simulink model "SecRwRtStLtwdRtwdIsPosChk"  (R2018b)
settings: Solver=FixedStepDiscrete  StartTime=0.0  StopTime=10.0  FixedStep=0.01  RelTol=1e-3
undefined symbols (not defined in the file or in its folder): KeSMSuSecRwStLwdRwdPosDelta_Val, KeSMSuSecRwStLwdRwdPosTolr_Val
libraries: StIsPosChkLib x9, simulink x5
settings Model: Creator=sn2xws  LastModifiedBy=sn2xws
settings DataIOCC: SaveFormat=StructureWithTime
settings OptimizationCC: DefaultParameterBehavior=Inlined  EnhancedBackFolding=on  PassReuseOutputArgsAs=Individual arguments  ZeroExternalMemoryAtStartup=off  ZeroInternalMemoryAtStartup=off  OptimizeBlockOrder=speed  DifferentSizesBufferReuse=on  OptimizationCustomize=off
settings DebuggingCC: ParameterTunabilityLossMsg=error
settings ModelReferenceCC: ModelReferenceNumInstancesAllowed=Single
settings SFSimCC: MATLABDynamicMemAlloc=off
settings RTWCC: SystemTargetFile=autosar.tlc  GenCodeOnly=on  TemplateMakefile=ert_default_tmf  Description=AUTOSAR  GenerateReport=on  IncludeHyperlinkInReport=on  LaunchReport=on  GenerateTraceInfo=on  GenerateTraceReport=on  GenerateTraceReportSl=on  GenerateTraceReportSf=on  GenerateTraceReportEml=on
settings CodeAppCC: ForceParamTrailComments=on  IgnoreCustomStorageClasses=off  OperatorAnnotations=on  SimulinkDataObjDesc=on  SFDataObjDesc=on  InsertBlockDesc=on
settings STFCustomTargetCC: TargetLangStandard=C99 (ISO)  MultiwordLength=256  ParMdlRefBuildCompliant=on  CompOptLevelCompliant=on  IncludeMdlTerminateFcn=off  CombineOutputUpdateFcns=on  SuppressErrorStatus=on  ERTCustomFileBanners=on  SupportNonFinite=off  SupportComplex=off  SupportContinuousTime=off  SupportNonInlinedSFcns=off  RemoveResetFunc=on  MATLABClassNameForMDSCustomization=Simulink.SoftwareTarget.ERTCustomization  AutosarCompliant=on  UseToolchainInfoCompliant=on  LookupTableObjectStructAxisOrder=2,1,3,4,...  LUTObjectStructOrderEvenSpacing=Size,Table,Breakpoints  SystemTargetFile=autosar.tlc
settings ERTTargetCC: TargetLangStandard=C99 (ISO)  ConcurrentExecutionCompliant=off  IncludeMdlTerminateFcn=off  SuppressErrorStatus=on  SupportNonFinite=off  SupportComplex=off  ModelStepFunctionPrototypeControlCompliant=off  CPPClassGenCompliant=off  AutosarCompliant=on  LookupTableObjectStructAxisOrder=2,1,3,4,...  LUTObjectStructOrderEvenSpacing=Size,Table,Breakpoints  InlinedParameterPlacement=NonHierarchical  ERTCustomFileTemplate=example_file_process.tlc  ERTFilePackagingFormat=Compact

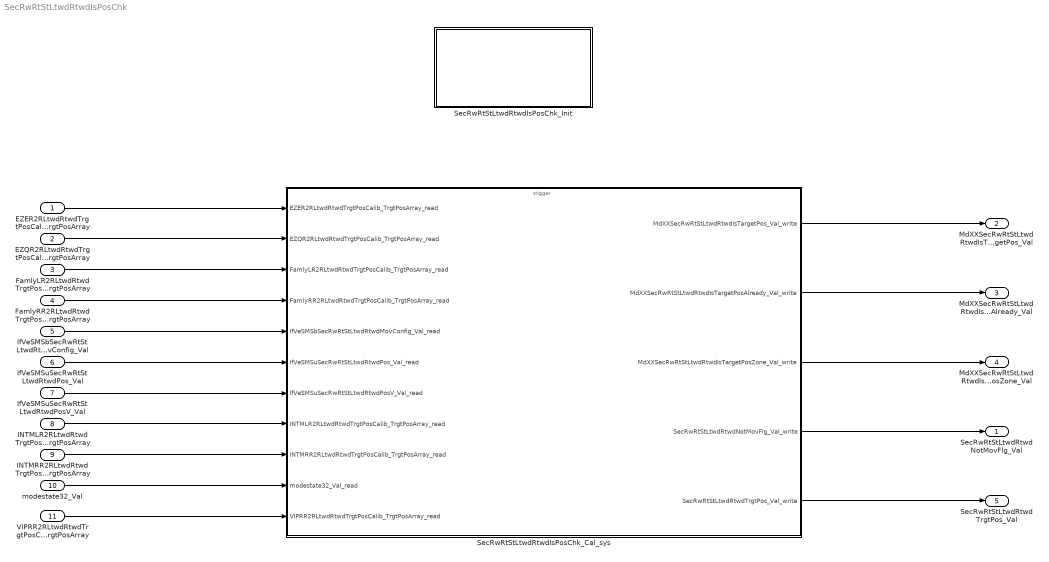
== system SecRwRtStLtwdRtwdIsPosChk ==
  EZER2RLtwdRtwdTrgtPosCalib_TrgtPosArray : Inport  Description=|  OutDataTypeStr=uint16  PortDimensions=3
      | 0:Pos
      | 1:Max
      | 2:Min
  EZQR2RLtwdRtwdTrgtPosCalib_TrgtPosArray : Inport  Description=|  Port=2  OutDataTypeStr=uint16  PortDimensions=3
      | 0:Pos
      | 1:Max
      | 2:Min
  FamlyLR2RLtwdRtwdTrgtPosCalib_TrgtPosArray : Inport  Description=|  Port=3  OutDataTypeStr=uint16  PortDimensions=3
      | 0:Pos
      | 1:Max
      | 2:Min
  FamlyRR2RLtwdRtwdTrgtPosCalib_TrgtPosArray : Inport  Description=|  Port=4  OutDataTypeStr=uint16  PortDimensions=3
      | 0:Pos
      | 1:Max
      | 2:Min
  IfVeSMSbSecRwRtStLtwdRtwdMovConfig_Val : Inport  Port=5  OutDataTypeStr=boolean  PortDimensions=1
  IfVeSMSuSecRwRtStLtwdRtwdPos_Val : Inport  Port=6  OutDataTypeStr=uint16  PortDimensions=1
  IfVeSMSuSecRwRtStLtwdRtwdPosV_Val : Inport  Port=7  OutDataTypeStr=boolean  PortDimensions=1
  INTMLR2RLtwdRtwdTrgtPosCalib_TrgtPosArray : Inport  Description=|  Port=8  OutDataTypeStr=uint16  PortDimensions=3
      | 0:Pos
      | 1:Max
      | 2:Min
  INTMRR2RLtwdRtwdTrgtPosCalib_TrgtPosArray : Inport  Description=|  Port=9  OutDataTypeStr=uint16  PortDimensions=3
      | 0:Pos
      | 1:Max
      | 2:Min
  modestate32_Val : Inport  Port=10  OutDataTypeStr=uint32  PortDimensions=1
  VIPRR2RLtwdRtwdTrgtPosCalib_TrgtPosArray : Inport  Description=|  Port=11  OutDataTypeStr=uint16  PortDimensions=3
      | 0:Pos
      | 1:Max
      | 2:Min
  SecRwRtStLtwdRtwdIsPosChk_Cal_sys : Subsystem
  SecRwRtStLtwdRtwdIsPosChk_Init : Subsystem
  SecRwRtStLtwdRtwdNotMovFlg_Val : Outport  OutDataTypeStr=boolean  PortDimensions=1
  MdXXSecRwRtStLtwdRtwdIsTargetPos_Val : Outport  Port=2  OutDataTypeStr=uint32  PortDimensions=1
  MdXXSecRwRtStLtwdRtwdIsTargetPosAlready_Val : Outport  Port=3  OutDataTypeStr=uint32  PortDimensions=1
  MdXXSecRwRtStLtwdRtwdIsTargetPosZone_Val : Outport  Port=4  OutDataTypeStr=uint32  PortDimensions=1
  SecRwRtStLtwdRtwdTrgtPos_Val : Outport  Port=5  OutDataTypeStr=uint16  PortDimensions=1
  wires:
  EZER2RLtwdRtwdTrgtPosCalib_TrgtPosArray/1 -> SecRwRtStLtwdRtwdIsPosChk_Cal_sys/1(EZER2RLtwdRtwdTrgtPosCalib_TrgtPosArray_read)
  EZQR2RLtwdRtwdTrgtPosCalib_TrgtPosArray/1 -> SecRwRtStLtwdRtwdIsPosChk_Cal_sys/2(EZQR2RLtwdRtwdTrgtPosCalib_TrgtPosArray_read)
  FamlyLR2RLtwdRtwdTrgtPosCalib_TrgtPosArray/1 -> SecRwRtStLtwdRtwdIsPosChk_Cal_sys/3(FamlyLR2RLtwdRtwdTrgtPosCalib_TrgtPosArray_read)
  FamlyRR2RLtwdRtwdTrgtPosCalib_TrgtPosArray/1 -> SecRwRtStLtwdRtwdIsPosChk_Cal_sys/4(FamlyRR2RLtwdRtwdTrgtPosCalib_TrgtPosArray_read)
  IfVeSMSbSecRwRtStLtwdRtwdMovConfig_Val/1 -> SecRwRtStLtwdRtwdIsPosChk_Cal_sys/5(IfVeSMSbSecRwRtStLtwdRtwdMovConfig_Val_read)
  IfVeSMSuSecRwRtStLtwdRtwdPos_Val/1 -> SecRwRtStLtwdRtwdIsPosChk_Cal_sys/6(IfVeSMSuSecRwRtStLtwdRtwdPos_Val_read)
  IfVeSMSuSecRwRtStLtwdRtwdPosV_Val/1 -> SecRwRtStLtwdRtwdIsPosChk_Cal_sys/7(IfVeSMSuSecRwRtStLtwdRtwdPosV_Val_read)
  INTMLR2RLtwdRtwdTrgtPosCalib_TrgtPosArray/1 -> SecRwRtStLtwdRtwdIsPosChk_Cal_sys/8(INTMLR2RLtwdRtwdTrgtPosCalib_TrgtPosArray_read)
  INTMRR2RLtwdRtwdTrgtPosCalib_TrgtPosArray/1 -> SecRwRtStLtwdRtwdIsPosChk_Cal_sys/9(INTMRR2RLtwdRtwdTrgtPosCalib_TrgtPosArray_read)
  modestate32_Val/1 -> SecRwRtStLtwdRtwdIsPosChk_Cal_sys/10(modestate32_Val_read)
  VIPRR2RLtwdRtwdTrgtPosCalib_TrgtPosArray/1 -> SecRwRtStLtwdRtwdIsPosChk_Cal_sys/11(VIPRR2RLtwdRtwdTrgtPosCalib_TrgtPosArray_read)
  SecRwRtStLtwdRtwdIsPosChk_Cal_sys/1(MdXXSecRwRtStLtwdRtwdIsTargetPos_Val_write) -> MdXXSecRwRtStLtwdRtwdIsTargetPos_Val/1
  SecRwRtStLtwdRtwdIsPosChk_Cal_sys/2(MdXXSecRwRtStLtwdRtwdIsTargetPosAlready_Val_write) -> MdXXSecRwRtStLtwdRtwdIsTargetPosAlready_Val/1
  SecRwRtStLtwdRtwdIsPosChk_Cal_sys/3(MdXXSecRwRtStLtwdRtwdIsTargetPosZone_Val_write) -> MdXXSecRwRtStLtwdRtwdIsTargetPosZone_Val/1
  SecRwRtStLtwdRtwdIsPosChk_Cal_sys/4(SecRwRtStLtwdRtwdNotMovFlg_Val_write) -> SecRwRtStLtwdRtwdNotMovFlg_Val/1
  SecRwRtStLtwdRtwdIsPosChk_Cal_sys/5(SecRwRtStLtwdRtwdTrgtPos_Val_write) -> SecRwRtStLtwdRtwdTrgtPos_Val/1

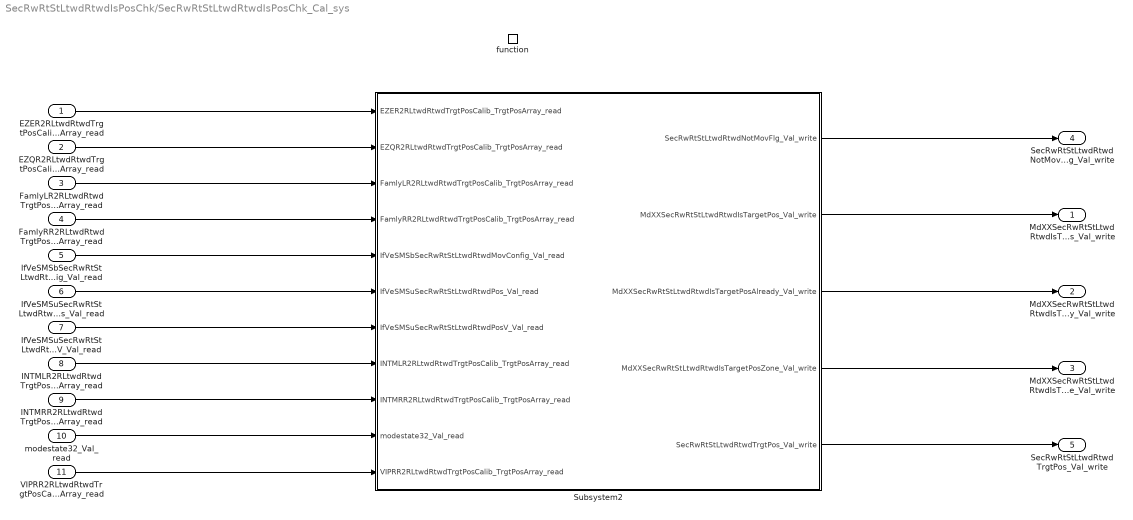
== system SecRwRtStLtwdRtwdIsPosChk/SecRwRtStLtwdRtwdIsPosChk_Cal_sys ==
  EZER2RLtwdRtwdTrgtPosCalib_TrgtPosArray_read : Inport
  EZQR2RLtwdRtwdTrgtPosCalib_TrgtPosArray_read : Inport  Port=2
  FamlyLR2RLtwdRtwdTrgtPosCalib_TrgtPosArray_read : Inport  Port=3
  FamlyRR2RLtwdRtwdTrgtPosCalib_TrgtPosArray_read : Inport  Port=4
  IfVeSMSbSecRwRtStLtwdRtwdMovConfig_Val_read : Inport  Port=5
  IfVeSMSuSecRwRtStLtwdRtwdPos_Val_read : Inport  Port=6
  IfVeSMSuSecRwRtStLtwdRtwdPosV_Val_read : Inport  Port=7
  INTMLR2RLtwdRtwdTrgtPosCalib_TrgtPosArray_read : Inport  Port=8
  INTMRR2RLtwdRtwdTrgtPosCalib_TrgtPosArray_read : Inport  Port=9
  modestate32_Val_read : Inport  Port=10
  VIPRR2RLtwdRtwdTrgtPosCalib_TrgtPosArray_read : Inport  Port=11
  function : TriggerPort  TriggerType=function-call  IsSimulinkFunction=on  FunctionName=SecRwRtStLtwdRtwdIsPosChk_Cal  VariantControl=(inherit)
  Subsystem2 : Subsystem
  MdXXSecRwRtStLtwdRtwdIsTargetPos_Val_write : Outport
      settings: EnsureOutportIsVirtual=on
  MdXXSecRwRtStLtwdRtwdIsTargetPosAlready_Val_write : Outport  Port=2
      settings: EnsureOutportIsVirtual=on
  MdXXSecRwRtStLtwdRtwdIsTargetPosZone_Val_write : Outport  Port=3
      settings: EnsureOutportIsVirtual=on
  SecRwRtStLtwdRtwdNotMovFlg_Val_write : Outport  Port=4
      settings: EnsureOutportIsVirtual=on
  SecRwRtStLtwdRtwdTrgtPos_Val_write : Outport  Port=5
      settings: EnsureOutportIsVirtual=on
  wires:
  EZER2RLtwdRtwdTrgtPosCalib_TrgtPosArray_read/1 -> Subsystem2/1(EZER2RLtwdRtwdTrgtPosCalib_TrgtPosArray_read)
  EZQR2RLtwdRtwdTrgtPosCalib_TrgtPosArray_read/1 -> Subsystem2/2(EZQR2RLtwdRtwdTrgtPosCalib_TrgtPosArray_read)
  FamlyLR2RLtwdRtwdTrgtPosCalib_TrgtPosArray_read/1 -> Subsystem2/3(FamlyLR2RLtwdRtwdTrgtPosCalib_TrgtPosArray_read)
  FamlyRR2RLtwdRtwdTrgtPosCalib_TrgtPosArray_read/1 -> Subsystem2/4(FamlyRR2RLtwdRtwdTrgtPosCalib_TrgtPosArray_read)
  IfVeSMSbSecRwRtStLtwdRtwdMovConfig_Val_read/1 -> Subsystem2/5(IfVeSMSbSecRwRtStLtwdRtwdMovConfig_Val_read)
  IfVeSMSuSecRwRtStLtwdRtwdPos_Val_read/1 -> Subsystem2/6(IfVeSMSuSecRwRtStLtwdRtwdPos_Val_read)
  IfVeSMSuSecRwRtStLtwdRtwdPosV_Val_read/1 -> Subsystem2/7(IfVeSMSuSecRwRtStLtwdRtwdPosV_Val_read)
  INTMLR2RLtwdRtwdTrgtPosCalib_TrgtPosArray_read/1 -> Subsystem2/8(INTMLR2RLtwdRtwdTrgtPosCalib_TrgtPosArray_read)
  INTMRR2RLtwdRtwdTrgtPosCalib_TrgtPosArray_read/1 -> Subsystem2/9(INTMRR2RLtwdRtwdTrgtPosCalib_TrgtPosArray_read)
  modestate32_Val_read/1 -> Subsystem2/10(modestate32_Val_read)
  VIPRR2RLtwdRtwdTrgtPosCalib_TrgtPosArray_read/1 -> Subsystem2/11(VIPRR2RLtwdRtwdTrgtPosCalib_TrgtPosArray_read)
  Subsystem2/1(SecRwRtStLtwdRtwdNotMovFlg_Val_write) -> SecRwRtStLtwdRtwdNotMovFlg_Val_write/1
  Subsystem2/2(MdXXSecRwRtStLtwdRtwdIsTargetPos_Val_write) -> MdXXSecRwRtStLtwdRtwdIsTargetPos_Val_write/1
  Subsystem2/3(MdXXSecRwRtStLtwdRtwdIsTargetPosAlready_Val_write) -> MdXXSecRwRtStLtwdRtwdIsTargetPosAlready_Val_write/1
  Subsystem2/4(MdXXSecRwRtStLtwdRtwdIsTargetPosZone_Val_write) -> MdXXSecRwRtStLtwdRtwdIsTargetPosZone_Val_write/1
  Subsystem2/5(SecRwRtStLtwdRtwdTrgtPos_Val_write) -> SecRwRtStLtwdRtwdTrgtPos_Val_write/1

== system SecRwRtStLtwdRtwdIsPosChk/SecRwRtStLtwdRtwdIsPosChk_Init ==
  Event Listener : EventListener  EventName=reset

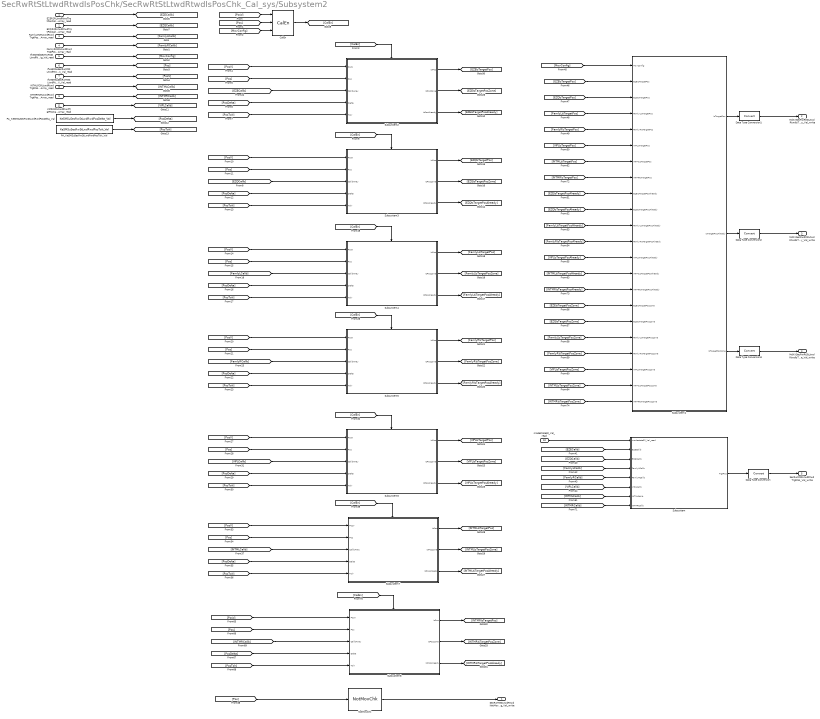
== system SecRwRtStLtwdRtwdIsPosChk/SecRwRtStLtwdRtwdIsPosChk_Cal_sys/Subsystem2 ==
  EZER2RLtwdRtwdTrgtPosCalib_TrgtPosArray_read : Inport
  EZQR2RLtwdRtwdTrgtPosCalib_TrgtPosArray_read : Inport  Port=2
  FamlyLR2RLtwdRtwdTrgtPosCalib_TrgtPosArray_read : Inport  Port=3
  FamlyRR2RLtwdRtwdTrgtPosCalib_TrgtPosArray_read : Inport  Port=4
  IfVeSMSbSecRwRtStLtwdRtwdMovConfig_Val_read : Inport  Port=5
  IfVeSMSuSecRwRtStLtwdRtwdPos_Val_read : Inport  Port=6
  IfVeSMSuSecRwRtStLtwdRtwdPosV_Val_read : Inport  Port=7
  INTMLR2RLtwdRtwdTrgtPosCalib_TrgtPosArray_read : Inport  Port=8
  INTMRR2RLtwdRtwdTrgtPosCalib_TrgtPosArray_read : Inport  Port=9
  modestate32_Val_read : Inport  Port=10
  VIPRR2RLtwdRtwdTrgtPosCalib_TrgtPosArray_read : Inport  Port=11
  CalEn : StIsPosChkLib/CalEn  SystemSampleTime=-1
  Data Type Conversion{,1..3} (4 alike) : DataTypeConversion
  NotMovChk : StIsPosChkLib/NotMovChk  SystemSampleTime=-1
  PA_KeSMSuSecRwStLwdRwdPosDelta_Val : Constant  Value=KeSMSuSecRwStLwdRwdPosDelta_Val
  PA_KeSMSuSecRwStLwdRwdPosTolr_Val : Constant  Value=KeSMSuSecRwStLwdRwdPosTolr_Val
  Subsystem : Subsystem
  Subsystem1 : Subsystem
  Subsystem2 : Subsystem
  Subsystem3 : Subsystem
  Subsystem4 : Subsystem
  Subsystem5 : Subsystem
  Subsystem6 : Subsystem
  Subsystem7 : Subsystem
  Subsystem8 : Subsystem
  SecRwRtStLtwdRtwdNotMovFlg_Val_write : Outport
      settings: EnsureOutportIsVirtual=on
  MdXXSecRwRtStLtwdRtwdIsTargetPos_Val_write : Outport  Port=2
      settings: EnsureOutportIsVirtual=on
  MdXXSecRwRtStLtwdRtwdIsTargetPosAlready_Val_write : Outport  Port=3
      settings: EnsureOutportIsVirtual=on
  MdXXSecRwRtStLtwdRtwdIsTargetPosZone_Val_write : Outport  Port=4
      settings: EnsureOutportIsVirtual=on
  SecRwRtStLtwdRtwdTrgtPos_Val_write : Outport  Port=5
      settings: EnsureOutportIsVirtual=on
  wires:
  [PosTolr] -> Subsystem7/5(Tolr)
  Subsystem6/1(IsPos) -> [VIPLIsTargetPos]
  [INTMRIsTargetPosAlready] -> Subsystem1/15(INTMRIsTargetPosAlready)
  [Pos] -> Subsystem6/2(Pos)
  CalEn/1 -> [CalEn]
  [CalEn] -> Subsystem8/Enable
  [FamlyLIsTargetPos] -> Subsystem1/4(FamlyLIsTargetPos)
  [PosTolr] -> Subsystem4/5(Tolr)
  EZQR2RLtwdRtwdTrgtPosCalib_TrgtPosArray_read/1 -> [EZQCalib]
  [EZQIsTargetPosZone] -> Subsystem1/17(EZQIsTargetPosZone)
  FamlyLR2RLtwdRtwdTrgtPosCalib_TrgtPosArray_read/1 -> [FamlyLCalib]
  INTMLR2RLtwdRtwdTrgtPosCalib_TrgtPosArray_read/1 -> [INTMLCalib]
  [PosTolr] -> Subsystem2/5(Tolr)
  EZER2RLtwdRtwdTrgtPosCalib_TrgtPosArray_read/1 -> [EZECalib]
  [PosDelta] -> Subsystem2/4(Delta)
  [VIPLCalib] -> Subsystem6/3(CalibArray)
  [VIPLIsTargetPosAlready] -> Subsystem1/13(VIPLIsTargetPosAlready)
  [FamlyRIsTargetPosZone] -> Subsystem1/19(FamlyRIsTargetPosZone)
  VIPRR2RLtwdRtwdTrgtPosCalib_TrgtPosArray_read/1 -> [VIPLCalib]
  Subsystem5/3(IsPosAlready) -> [FamlyRIsTargetPosAlready]
  PA_KeSMSuSecRwStLwdRwdPosDelta_Val/1 -> [PosDelta]
  Subsystem3/2(IsPosZone) -> [EZQIsTargetPosZone]
  [PosV] -> Subsystem2/1(PosV)
  [PosV] -> Subsystem6/1(PosV)
  [PosDelta] -> Subsystem5/4(Delta)
  [EZEIsTargetPos] -> Subsystem1/2(EZEIsTargetPos)
  Subsystem8/1(IsPos) -> [INTMRIsTargetPos]
  [CalEn] -> Subsystem7/Enable
  [Pos] -> Subsystem4/2(Pos)
  [Pos] -> Subsystem7/2(Pos)
  [FamlyLCalib] -> Subsystem/4(FamlyLCalib)
  Subsystem3/1(IsPos) -> [EZQIsTargetPos]
  [VIPLIsTargetPosZone] -> Subsystem1/20(VIPLIsTargetPosZone)
  [PosDelta] -> Subsystem7/4(Delta)
  [Pos] -> Subsystem2/2(Pos)
  NotMovChk/1 -> SecRwRtStLtwdRtwdNotMovFlg_Val_write/1
  [EZEIsTargetPosAlready] -> Subsystem1/9(EZEIsTargetPosAlready)
  Subsystem5/2(IsPosZone) -> [FamlyRIsTargetPosZone]
  [INTMRCalib] -> Subsystem/8(INTMRCalib)
  [INTMLIsTargetPos] -> Subsystem1/7(INTMLIsTargetPos)
  [INTMLCalib] -> Subsystem/7(INTMLCalib)
  Subsystem4/3(IsPosAlready) -> [FamlyLIsTargetPosAlready]
  [Pos] -> NotMovChk/1
  Data Type Conversion2/1 -> MdXXSecRwRtStLtwdRtwdIsTargetPosAlready_Val_write/1
  [PosDelta] -> Subsystem8/4(Delta)
  Subsystem5/1(IsPos) -> [FamlyRIsTargetPos]
  Subsystem1/2(IsTargetPosAlready) -> Data Type Conversion2/1
  Subsystem7/1(IsPos) -> [INTMLIsTargetPos]
  IfVeSMSbSecRwRtStLtwdRtwdMovConfig_Val_read/1 -> [MovConfig]
  [INTMRCalib] -> Subsystem8/3(CalibArray)
  [EZECalib] -> Subsystem2/3(CalibArray)
  [PosTolr] -> Subsystem6/5(Tolr)
  [PosV] -> CalEn/1
  [EZQIsTargetPosAlready] -> Subsystem1/10(EZQIsTargetPosAlready)
  [EZQCalib] -> Subsystem3/3(CalibArray)
  Subsystem2/1(IsPos) -> [EZEIsTargetPos]
  Subsystem/1(TrgtPos) -> Data Type Conversion/1
  [EZQCalib] -> Subsystem/3(EZQCalib)
  [FamlyLIsTargetPosAlready] -> Subsystem1/11(FamlyLIsTargetPosAlready)
  Data Type Conversion3/1 -> MdXXSecRwRtStLtwdRtwdIsTargetPosZone_Val_write/1
  [PosV] -> Subsystem5/1(PosV)
  [VIPLIsTargetPos] -> Subsystem1/6(VIPLIsTargetPos)
  FamlyRR2RLtwdRtwdTrgtPosCalib_TrgtPosArray_read/1 -> [FamlyRCalib]
  [EZEIsTargetPosZone] -> Subsystem1/16(EZEIsTargetPosZone)
  [PosTolr] -> Subsystem8/5(Tolr)
  Subsystem6/2(IsPosZone) -> [VIPLIsTargetPosZone]
  [VIPLCalib] -> Subsystem/6(VIPLCalib)
  Subsystem4/2(IsPosZone) -> [FamlyLIsTargetPosZone]
  [PosTolr] -> Subsystem3/5(Tolr)
  [FamlyLIsTargetPosZone] -> Subsystem1/18(FamlyLIsTargetPosZone)
  [EZECalib] -> Subsystem/2(EZECalib)
  [FamlyRIsTargetPosAlready] -> Subsystem1/12(FamlyRIsTargetPosAlready)
  Subsystem6/3(IsPosAlready) -> [VIPLIsTargetPosAlready]
  [CalEn] -> Subsystem6/Enable
  [FamlyRCalib] -> Subsystem5/3(CalibArray)
  [PosV] -> Subsystem4/1(PosV)
  [PosDelta] -> Subsystem4/4(Delta)
  [PosV] -> Subsystem8/1(PosV)
  [Pos] -> Subsystem8/2(Pos)
  [INTMLIsTargetPosAlready] -> Subsystem1/14(INTMLIsTargetPosAlready)
  INTMRR2RLtwdRtwdTrgtPosCalib_TrgtPosArray_read/1 -> [INTMRCalib]
  [Pos] -> Subsystem5/2(Pos)
  IfVeSMSuSecRwRtStLtwdRtwdPos_Val_read/1 -> [Pos]
  Subsystem7/3(IsPosAlready) -> [INTMLIsTargetPosAlready]
  [FamlyRIsTargetPos] -> Subsystem1/5(FamlyRIsTargetPos)
  Subsystem3/3(IsPosAlready) -> [EZQIsTargetPosAlready]
  [EZQIsTargetPos] -> Subsystem1/3(EZQIsTargetPos)
  Data Type Conversion1/1 -> MdXXSecRwRtStLtwdRtwdIsTargetPos_Val_write/1
  PA_KeSMSuSecRwStLwdRwdPosTolr_Val/1 -> [PosTolr]
  [INTMRIsTargetPos] -> Subsystem1/8(INTMRIsTargetPos)
  [FamlyLCalib] -> Subsystem4/3(CalibArray)
  [PosDelta] -> Subsystem6/4(Delta)
  Subsystem1/1(IsTargetPos) -> Data Type Conversion1/1
  [MovConfig] -> Subsystem1/1(MovConfig)
  [MovConfig] -> CalEn/3
  [CalEn] -> Subsystem2/Enable
  IfVeSMSuSecRwRtStLtwdRtwdPosV_Val_read/1 -> [PosV]
  [Pos] -> CalEn/2
  Subsystem7/2(IsPosZone) -> [INTMLIsTargetPosZone]
  [PosV] -> Subsystem3/1(PosV)
  [PosTolr] -> Subsystem5/5(Tolr)
  Subsystem8/2(IsPosZone) -> [INTMRIsTargetPosZone]
  [Pos] -> Subsystem3/2(Pos)
  [FamlyRCalib] -> Subsystem/5(FamlyRCalib)
  [CalEn] -> Subsystem3/Enable
  [INTMLCalib] -> Subsystem7/3(CalibArray)
  Subsystem1/3(IsTargetPosZone) -> Data Type Conversion3/1
  [PosDelta] -> Subsystem3/4(Delta)
  Subsystem8/3(IsPosAlready) -> [INTMRIsTargetPosAlready]
  Subsystem2/3(IsPosAlready) -> [EZEIsTargetPosAlready]
  [CalEn] -> Subsystem5/Enable
  [CalEn] -> Subsystem4/Enable
  [INTMRIsTargetPosZone] -> Subsystem1/22(INTMRIsTargetPosZone)
  [INTMLIsTargetPosZone] -> Subsystem1/21(INTMLIsTargetPosZone)
  Subsystem2/2(IsPosZone) -> [EZEIsTargetPosZone]
  Subsystem4/1(IsPos) -> [FamlyLIsTargetPos]
  [PosV] -> Subsystem7/1(PosV)
  modestate32_Val_read/1 -> Subsystem/1(modestate32_Val_read)
  Data Type Conversion/1 -> SecRwRtStLtwdRtwdTrgtPos_Val_write/1

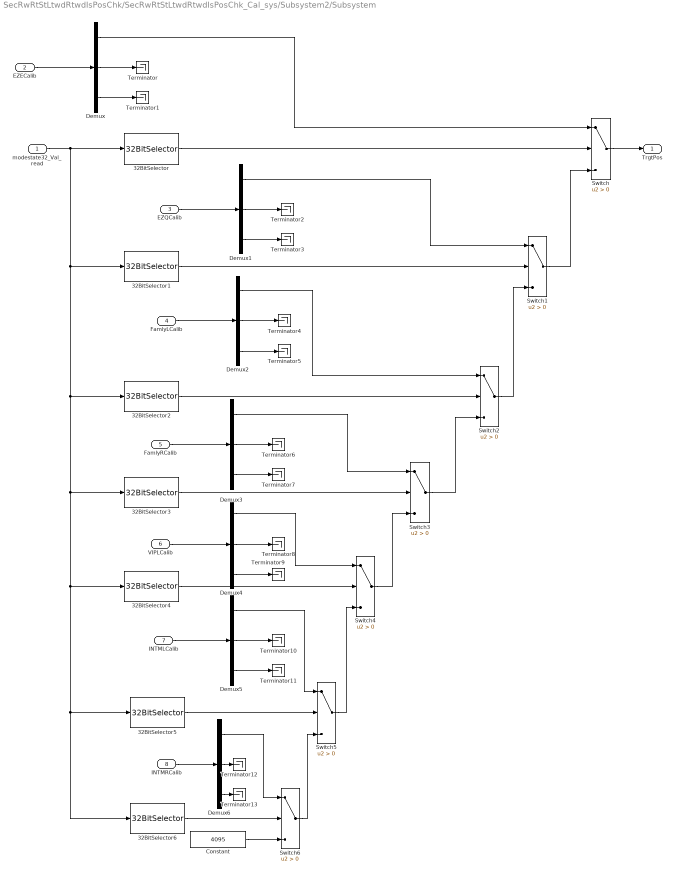
== system SecRwRtStLtwdRtwdIsPosChk/SecRwRtStLtwdRtwdIsPosChk_Cal_sys/Subsystem2/Subsystem ==
  modestate32_Val_read : Inport
  EZECalib : Inport  Port=2
  EZQCalib : Inport  Port=3
  FamlyLCalib : Inport  Port=4
  FamlyRCalib : Inport  Port=5
  VIPLCalib : Inport  Port=6
  INTMLCalib : Inport  Port=7
  INTMRCalib : Inport  Port=8
  32BitSelector : StIsPosChkLib/32BitSelector  BitNum=0
  32BitSelector1 : StIsPosChkLib/32BitSelector  BitNum=3
  32BitSelector2 : StIsPosChkLib/32BitSelector  BitNum=6
  32BitSelector3 : StIsPosChkLib/32BitSelector  BitNum=5
  32BitSelector4 : StIsPosChkLib/32BitSelector  BitNum=11
  32BitSelector5 : StIsPosChkLib/32BitSelector  BitNum=4
  32BitSelector6 : StIsPosChkLib/32BitSelector  BitNum=19
  Constant : Constant  Value=4095  OutDataTypeStr=uint16
  Demux{,1..6} (7 alike) : Demux  Outputs=3
  Switch{,1..6} (7 alike) : Switch  Criteria=u2 > Threshold
  Terminator{,1..13} (14 alike) : Terminator
  TrgtPos : Outport
      settings: EnsureOutportIsVirtual=on
  wires:
  32BitSelector/1 -> Switch/2
  modestate32_Val_read/1 -> 32BitSelector2/1, 32BitSelector6/1, 32BitSelector5/1, 32BitSelector4/1, 32BitSelector3/1, 32BitSelector1/1, 32BitSelector/1
  Demux/1 -> Switch/1
  Demux/3 -> Terminator1/1
  Demux/2 -> Terminator/1
  EZECalib/1 -> Demux/1
  EZQCalib/1 -> Demux1/1
  Demux1/2 -> Terminator2/1
  Demux1/3 -> Terminator3/1
  Demux1/1 -> Switch1/1
  Switch/1 -> TrgtPos/1
  Switch1/1 -> Switch/3
  32BitSelector1/1 -> Switch1/2
  Switch2/1 -> Switch1/3
  Switch3/1 -> Switch2/3
  Switch4/1 -> Switch3/3
  32BitSelector2/1 -> Switch2/2
  32BitSelector3/1 -> Switch3/2
  32BitSelector4/1 -> Switch4/2
  Demux2/1 -> Switch2/1
  Demux2/3 -> Terminator5/1
  Demux2/2 -> Terminator4/1
  FamlyLCalib/1 -> Demux2/1
  FamlyRCalib/1 -> Demux3/1
  Demux3/2 -> Terminator6/1
  Demux3/3 -> Terminator7/1
  Demux3/1 -> Switch3/1
  Demux4/1 -> Switch4/1
  Demux4/3 -> Terminator9/1
  Demux4/2 -> Terminator8/1
  VIPLCalib/1 -> Demux4/1
  INTMLCalib/1 -> Demux5/1
  Demux5/2 -> Terminator10/1
  Demux5/3 -> Terminator11/1
  Demux5/1 -> Switch5/1
  Switch5/1 -> Switch4/3
  32BitSelector5/1 -> Switch5/2
  Constant/1 -> Switch6/3
  32BitSelector6/1 -> Switch6/2
  INTMRCalib/1 -> Demux6/1
  Demux6/2 -> Terminator12/1
  Demux6/3 -> Terminator13/1
  Demux6/1 -> Switch6/1
  Switch6/1 -> Switch5/3

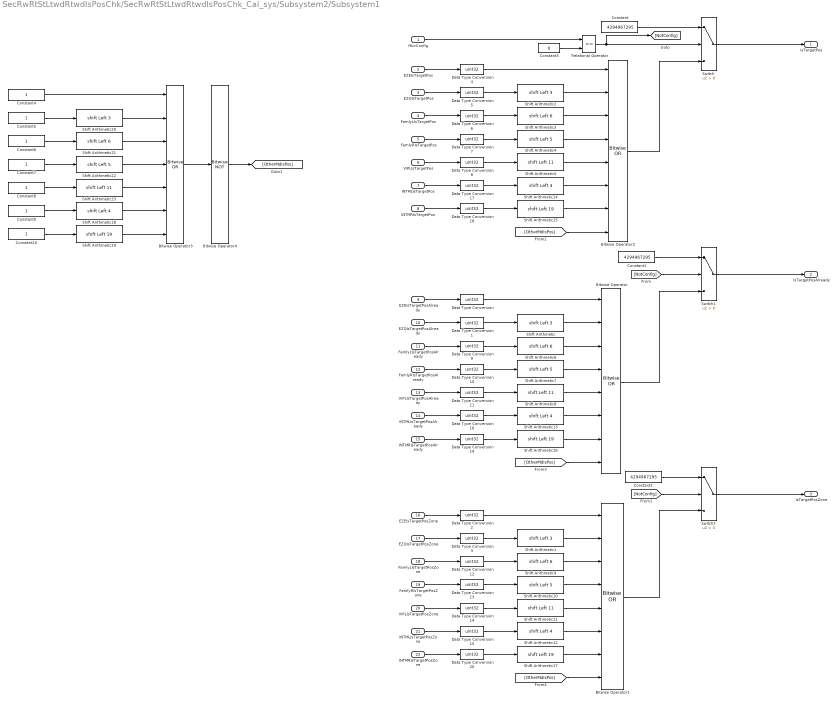
== system SecRwRtStLtwdRtwdIsPosChk/SecRwRtStLtwdRtwdIsPosChk_Cal_sys/Subsystem2/Subsystem1 ==
  MovConfig : Inport
  EZEIsTargetPos : Inport  Port=2
  EZQIsTargetPos : Inport  Port=3
  FamlyLIsTargetPos : Inport  Port=4
  FamlyRIsTargetPos : Inport  Port=5
  VIPLIsTargetPos : Inport  Port=6
  INTMLIsTargetPos : Inport  Port=7
  INTMRIsTargetPos : Inport  Port=8
  EZEIsTargetPosAlready : Inport  Port=9
  EZQIsTargetPosAlready : Inport  Port=10
  FamlyLIsTargetPosAlready : Inport  Port=11
  FamlyRIsTargetPosAlready : Inport  Port=12
  VIPLIsTargetPosAlready : Inport  Port=13
  INTMLIsTargetPosAlready : Inport  Port=14
  INTMRIsTargetPosAlready : Inport  Port=15
  EZEIsTargetPosZone : Inport  Port=16
  EZQIsTargetPosZone : Inport  Port=17
  FamlyLIsTargetPosZone : Inport  Port=18
  FamlyRIsTargetPosZone : Inport  Port=19
  VIPLIsTargetPosZone : Inport  Port=20
  INTMLIsTargetPosZone : Inport  Port=21
  INTMRIsTargetPosZone : Inport  Port=22
  Bitwise Operator : simulink/Logic and Bit Operations/Bitwise Operator  logicop=OR  UseBitMask=off  NumInputPorts=8  BitMask=bin2dec('11011001')  BitMaskRealWorld=Stored Integer
  Bitwise Operator1 : simulink/Logic and Bit Operations/Bitwise Operator  logicop=OR  UseBitMask=off  NumInputPorts=8  BitMask=bin2dec('11011001')  BitMaskRealWorld=Stored Integer
  Bitwise Operator2 : simulink/Logic and Bit Operations/Bitwise Operator  logicop=OR  UseBitMask=off  NumInputPorts=8  BitMask=bin2dec('11011001')  BitMaskRealWorld=Stored Integer
  Bitwise Operator3 : simulink/Logic and Bit Operations/Bitwise Operator  logicop=OR  UseBitMask=off  NumInputPorts=7  BitMask=bin2dec('11011001')  BitMaskRealWorld=Stored Integer
  Bitwise Operator4 : simulink/Logic and Bit Operations/Bitwise Operator  logicop=NOT  UseBitMask=off  BitMask=bin2dec('11011001')  BitMaskRealWorld=Stored Integer
  Constant : Constant  Value=4294967295  OutDataTypeStr=uint32
  Constant1 : Constant  Value=4294967295  OutDataTypeStr=uint32
  Constant{4..10} (7 alike) : Constant  OutDataTypeStr=uint32
  Constant2 : Constant  Value=4294967295  OutDataTypeStr=uint32
  Constant3 : Constant  Value=0  OutDataTypeStr=uint8
  Data Type Conversion{,1..20} (21 alike) : DataTypeConversion  OutDataTypeStr=uint32
  Relational Operator : RelationalOperator  Operator===  OutDataTypeStr=boolean  RndMeth=Simplest
  Shift Arithmetic{,1..2,20} (4 alike) : ArithShift  BitShiftNumber=3  BitShiftDirection=Left
  Shift Arithmetic{4,7,10,22} (4 alike) : ArithShift  BitShiftNumber=5  BitShiftDirection=Left
  Shift Arithmetic{5,8,11,23} (4 alike) : ArithShift  BitShiftNumber=11  BitShiftDirection=Left
  Shift Arithmetic{12..14,18} (4 alike) : ArithShift  BitShiftNumber=4  BitShiftDirection=Left
  Shift Arithmetic{15..17,19} (4 alike) : ArithShift  BitShiftNumber=19  BitShiftDirection=Left
  Shift Arithmetic{3,6,9,21} (4 alike) : ArithShift  BitShiftNumber=6  BitShiftDirection=Left
  Switch : Switch  Criteria=u2 > Threshold
  Switch1 : Switch  Criteria=u2 > Threshold
  Switch2 : Switch  Criteria=u2 > Threshold
  IsTargetPos : Outport
      settings: EnsureOutportIsVirtual=on
  IsTargetPosAlready : Outport  Port=2
      settings: EnsureOutportIsVirtual=on
  IsTargetPosZone : Outport  Port=3
      settings: EnsureOutportIsVirtual=on
  wires:
  Constant3/1 -> Relational Operator/2
  Constant/1 -> Switch/1
  Relational Operator/1 -> [NotConfig], Switch/2
  MovConfig/1 -> Relational Operator/1
  Switch/1 -> IsTargetPos/1
  [NotConfig] -> Switch1/2
  Constant1/1 -> Switch1/1
  Switch1/1 -> IsTargetPosAlready/1
  Switch2/1 -> IsTargetPosZone/1
  Constant2/1 -> Switch2/1
  [NotConfig] -> Switch2/2
  Data Type Conversion1/1 -> Shift Arithmetic/1
  Data Type Conversion/1 -> Bitwise Operator/1
  Shift Arithmetic/1 -> Bitwise Operator/2
  Shift Arithmetic1/1 -> Bitwise Operator1/2
  Data Type Conversion2/1 -> Bitwise Operator1/1
  Data Type Conversion3/1 -> Shift Arithmetic1/1
  Bitwise Operator1/1 -> Switch2/3
  Bitwise Operator/1 -> Switch1/3
  Shift Arithmetic2/1 -> Bitwise Operator2/2
  Data Type Conversion4/1 -> Bitwise Operator2/1
  Data Type Conversion5/1 -> Shift Arithmetic2/1
  Bitwise Operator2/1 -> Switch/3
  EZEIsTargetPos/1 -> Data Type Conversion4/1
  EZQIsTargetPos/1 -> Data Type Conversion5/1
  EZQIsTargetPosZone/1 -> Data Type Conversion3/1
  EZEIsTargetPosZone/1 -> Data Type Conversion2/1
  EZQIsTargetPosAlready/1 -> Data Type Conversion1/1
  EZEIsTargetPosAlready/1 -> Data Type Conversion/1
  Shift Arithmetic3/1 -> Bitwise Operator2/3
  Shift Arithmetic4/1 -> Bitwise Operator2/4
  Shift Arithmetic5/1 -> Bitwise Operator2/5
  Data Type Conversion7/1 -> Shift Arithmetic4/1
  Data Type Conversion6/1 -> Shift Arithmetic3/1
  Data Type Conversion8/1 -> Shift Arithmetic5/1
  FamlyLIsTargetPos/1 -> Data Type Conversion6/1
  FamlyRIsTargetPos/1 -> Data Type Conversion7/1
  VIPLIsTargetPos/1 -> Data Type Conversion8/1
  VIPLIsTargetPosAlready/1 -> Data Type Conversion11/1
  FamlyRIsTargetPosAlready/1 -> Data Type Conversion10/1
  FamlyLIsTargetPosAlready/1 -> Data Type Conversion9/1
  Data Type Conversion11/1 -> Shift Arithmetic8/1
  Data Type Conversion9/1 -> Shift Arithmetic6/1
  Data Type Conversion10/1 -> Shift Arithmetic7/1
  Shift Arithmetic8/1 -> Bitwise Operator/5
  Shift Arithmetic7/1 -> Bitwise Operator/4
  Shift Arithmetic6/1 -> Bitwise Operator/3
  Data Type Conversion14/1 -> Shift Arithmetic11/1
  Data Type Conversion13/1 -> Shift Arithmetic10/1
  VIPLIsTargetPosZone/1 -> Data Type Conversion14/1
  Shift Arithmetic10/1 -> Bitwise Operator1/4
  FamlyRIsTargetPosZone/1 -> Data Type Conversion13/1
  Shift Arithmetic9/1 -> Bitwise Operator1/3
  Shift Arithmetic11/1 -> Bitwise Operator1/5
  FamlyLIsTargetPosZone/1 -> Data Type Conversion12/1
  Data Type Conversion12/1 -> Shift Arithmetic9/1
  Shift Arithmetic12/1 -> Bitwise Operator1/6
  Data Type Conversion15/1 -> Shift Arithmetic12/1
  INTMLIsTargetPosZone/1 -> Data Type Conversion15/1
  Shift Arithmetic13/1 -> Bitwise Operator/6
  Data Type Conversion16/1 -> Shift Arithmetic13/1
  INTMLIsTargetPosAlready/1 -> Data Type Conversion16/1
  Shift Arithmetic14/1 -> Bitwise Operator2/6
  Data Type Conversion17/1 -> Shift Arithmetic14/1
  INTMLIsTargetPos/1 -> Data Type Conversion17/1
  INTMRIsTargetPos/1 -> Data Type Conversion18/1
  Data Type Conversion18/1 -> Shift Arithmetic15/1
  Shift Arithmetic15/1 -> Bitwise Operator2/7
  INTMRIsTargetPosAlready/1 -> Data Type Conversion19/1
  Data Type Conversion19/1 -> Shift Arithmetic16/1
  Shift Arithmetic16/1 -> Bitwise Operator/7
  INTMRIsTargetPosZone/1 -> Data Type Conversion20/1
  Data Type Conversion20/1 -> Shift Arithmetic17/1
  Shift Arithmetic17/1 -> Bitwise Operator1/7
  Shift Arithmetic19/1 -> Bitwise Operator3/7
  Constant10/1 -> Shift Arithmetic19/1
  Constant9/1 -> Shift Arithmetic18/1
  Shift Arithmetic18/1 -> Bitwise Operator3/6
  Constant8/1 -> Shift Arithmetic23/1
  Constant6/1 -> Shift Arithmetic21/1
  Constant7/1 -> Shift Arithmetic22/1
  Shift Arithmetic23/1 -> Bitwise Operator3/5
  Shift Arithmetic22/1 -> Bitwise Operator3/4
  Shift Arithmetic21/1 -> Bitwise Operator3/3
  Constant5/1 -> Shift Arithmetic20/1
  Constant4/1 -> Bitwise Operator3/1
  Shift Arithmetic20/1 -> Bitwise Operator3/2
  Bitwise Operator3/1 -> Bitwise Operator4/1
  Bitwise Operator4/1 -> [OtherMdIsPos]
  [OtherMdIsPos] -> Bitwise Operator2/8
  [OtherMdIsPos] -> Bitwise Operator/8
  [OtherMdIsPos] -> Bitwise Operator1/8

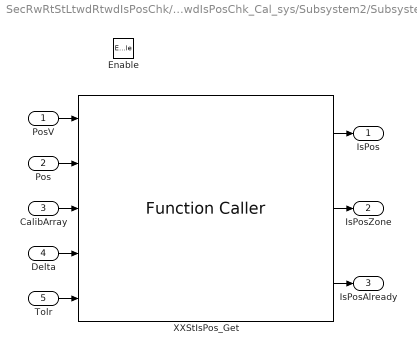
== system SecRwRtStLtwdRtwdIsPosChk/SecRwRtStLtwdRtwdIsPosChk_Cal_sys/Subsystem2/Subsystem2 ==
  PosV : Inport
  Pos : Inport  Port=2
  CalibArray : Inport  Port=3
  Delta : Inport  Port=4
  Tolr : Inport  Port=5
  Enable : EnablePort
  XXStIsPos_Get : FunctionCaller  FunctionPrototype=[IsPos,IsPosZone,IsPosAlready] = XXStIsPos_Get(PosV,Pos,CalibArray,Delta,Tolr)  InputArgumentSpecifications=boolean(true), uint16(1), uint16([1;1;1]), uint16(1), uint16(1)  OutputArgumentSpecifications=boolean(true), boolean(true), boolean(true)
  IsPos : Outport
  IsPosZone : Outport  Port=2
  IsPosAlready : Outport  Port=3
  wires:
  XXStIsPos_Get/1 -> IsPos/1
  Pos/1 -> XXStIsPos_Get/2
  Delta/1 -> XXStIsPos_Get/4
  XXStIsPos_Get/3 -> IsPosAlready/1
  PosV/1 -> XXStIsPos_Get/1
  CalibArray/1 -> XXStIsPos_Get/3
  Tolr/1 -> XXStIsPos_Get/5
  XXStIsPos_Get/2 -> IsPosZone/1

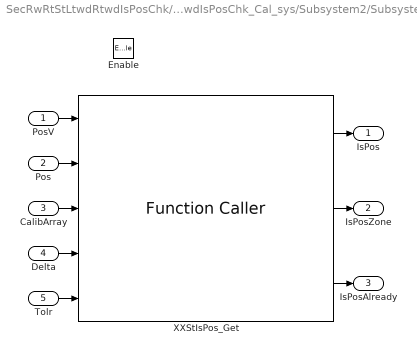
== system SecRwRtStLtwdRtwdIsPosChk/SecRwRtStLtwdRtwdIsPosChk_Cal_sys/Subsystem2/Subsystem3 ==
  PosV : Inport
  Pos : Inport  Port=2
  CalibArray : Inport  Port=3
  Delta : Inport  Port=4
  Tolr : Inport  Port=5
  Enable : EnablePort
  XXStIsPos_Get : FunctionCaller  FunctionPrototype=[IsPos,IsPosZone,IsPosAlready] = XXStIsPos_Get(PosV,Pos,CalibArray,Delta,Tolr)  InputArgumentSpecifications=boolean(true), uint16(1), uint16([1;1;1]), uint16(1), uint16(1)  OutputArgumentSpecifications=boolean(true), boolean(true), boolean(true)
  IsPos : Outport
  IsPosZone : Outport  Port=2
  IsPosAlready : Outport  Port=3
  wires:
  XXStIsPos_Get/1 -> IsPos/1
  Pos/1 -> XXStIsPos_Get/2
  Delta/1 -> XXStIsPos_Get/4
  XXStIsPos_Get/3 -> IsPosAlready/1
  PosV/1 -> XXStIsPos_Get/1
  CalibArray/1 -> XXStIsPos_Get/3
  Tolr/1 -> XXStIsPos_Get/5
  XXStIsPos_Get/2 -> IsPosZone/1

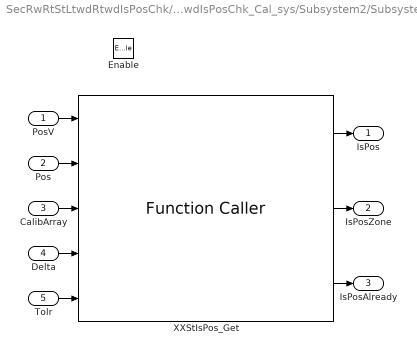
== system SecRwRtStLtwdRtwdIsPosChk/SecRwRtStLtwdRtwdIsPosChk_Cal_sys/Subsystem2/Subsystem4 ==
  PosV : Inport
  Pos : Inport  Port=2
  CalibArray : Inport  Port=3
  Delta : Inport  Port=4
  Tolr : Inport  Port=5
  Enable : EnablePort
  XXStIsPos_Get : FunctionCaller  FunctionPrototype=[IsPos,IsPosZone,IsPosAlready] = XXStIsPos_Get(PosV,Pos,CalibArray,Delta,Tolr)  InputArgumentSpecifications=boolean(true), uint16(1), uint16([1;1;1]), uint16(1), uint16(1)  OutputArgumentSpecifications=boolean(true), boolean(true), boolean(true)
  IsPos : Outport
  IsPosZone : Outport  Port=2
  IsPosAlready : Outport  Port=3
  wires:
  XXStIsPos_Get/1 -> IsPos/1
  Pos/1 -> XXStIsPos_Get/2
  Delta/1 -> XXStIsPos_Get/4
  XXStIsPos_Get/3 -> IsPosAlready/1
  PosV/1 -> XXStIsPos_Get/1
  CalibArray/1 -> XXStIsPos_Get/3
  Tolr/1 -> XXStIsPos_Get/5
  XXStIsPos_Get/2 -> IsPosZone/1

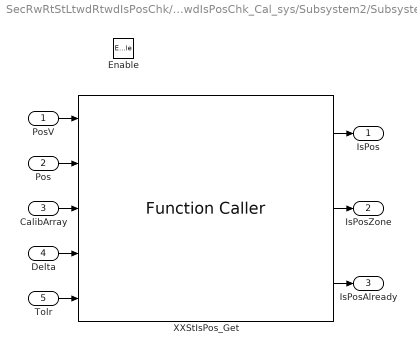
== system SecRwRtStLtwdRtwdIsPosChk/SecRwRtStLtwdRtwdIsPosChk_Cal_sys/Subsystem2/Subsystem5 ==
  PosV : Inport
  Pos : Inport  Port=2
  CalibArray : Inport  Port=3
  Delta : Inport  Port=4
  Tolr : Inport  Port=5
  Enable : EnablePort
  XXStIsPos_Get : FunctionCaller  FunctionPrototype=[IsPos,IsPosZone,IsPosAlready] = XXStIsPos_Get(PosV,Pos,CalibArray,Delta,Tolr)  InputArgumentSpecifications=boolean(true), uint16(1), uint16([1;1;1]), uint16(1), uint16(1)  OutputArgumentSpecifications=boolean(true), boolean(true), boolean(true)
  IsPos : Outport
  IsPosZone : Outport  Port=2
  IsPosAlready : Outport  Port=3
  wires:
  XXStIsPos_Get/1 -> IsPos/1
  Pos/1 -> XXStIsPos_Get/2
  Delta/1 -> XXStIsPos_Get/4
  XXStIsPos_Get/3 -> IsPosAlready/1
  PosV/1 -> XXStIsPos_Get/1
  CalibArray/1 -> XXStIsPos_Get/3
  Tolr/1 -> XXStIsPos_Get/5
  XXStIsPos_Get/2 -> IsPosZone/1

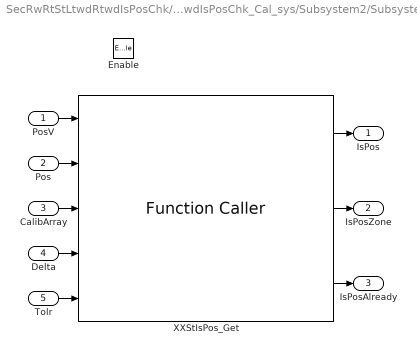
== system SecRwRtStLtwdRtwdIsPosChk/SecRwRtStLtwdRtwdIsPosChk_Cal_sys/Subsystem2/Subsystem6 ==
  PosV : Inport
  Pos : Inport  Port=2
  CalibArray : Inport  Port=3
  Delta : Inport  Port=4
  Tolr : Inport  Port=5
  Enable : EnablePort
  XXStIsPos_Get : FunctionCaller  FunctionPrototype=[IsPos,IsPosZone,IsPosAlready] = XXStIsPos_Get(PosV,Pos,CalibArray,Delta,Tolr)  InputArgumentSpecifications=boolean(true), uint16(1), uint16([1;1;1]), uint16(1), uint16(1)  OutputArgumentSpecifications=boolean(true), boolean(true), boolean(true)
  IsPos : Outport
  IsPosZone : Outport  Port=2
  IsPosAlready : Outport  Port=3
  wires:
  XXStIsPos_Get/1 -> IsPos/1
  Pos/1 -> XXStIsPos_Get/2
  Delta/1 -> XXStIsPos_Get/4
  XXStIsPos_Get/3 -> IsPosAlready/1
  PosV/1 -> XXStIsPos_Get/1
  CalibArray/1 -> XXStIsPos_Get/3
  Tolr/1 -> XXStIsPos_Get/5
  XXStIsPos_Get/2 -> IsPosZone/1

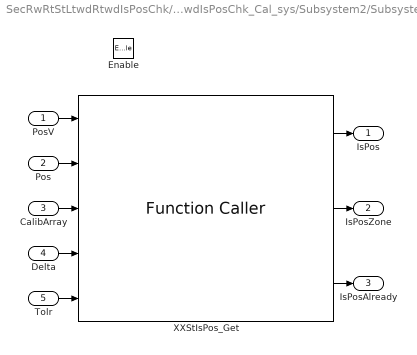
== system SecRwRtStLtwdRtwdIsPosChk/SecRwRtStLtwdRtwdIsPosChk_Cal_sys/Subsystem2/Subsystem7 ==
  PosV : Inport
  Pos : Inport  Port=2
  CalibArray : Inport  Port=3
  Delta : Inport  Port=4
  Tolr : Inport  Port=5
  Enable : EnablePort
  XXStIsPos_Get : FunctionCaller  FunctionPrototype=[IsPos,IsPosZone,IsPosAlready] = XXStIsPos_Get(PosV,Pos,CalibArray,Delta,Tolr)  InputArgumentSpecifications=boolean(true), uint16(1), uint16([1;1;1]), uint16(1), uint16(1)  OutputArgumentSpecifications=boolean(true), boolean(true), boolean(true)
  IsPos : Outport
  IsPosZone : Outport  Port=2
  IsPosAlready : Outport  Port=3
  wires:
  XXStIsPos_Get/1 -> IsPos/1
  Pos/1 -> XXStIsPos_Get/2
  Delta/1 -> XXStIsPos_Get/4
  XXStIsPos_Get/3 -> IsPosAlready/1
  PosV/1 -> XXStIsPos_Get/1
  CalibArray/1 -> XXStIsPos_Get/3
  Tolr/1 -> XXStIsPos_Get/5
  XXStIsPos_Get/2 -> IsPosZone/1

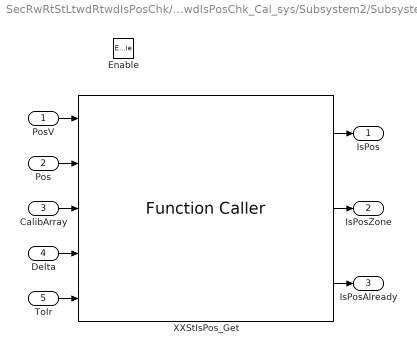
== system SecRwRtStLtwdRtwdIsPosChk/SecRwRtStLtwdRtwdIsPosChk_Cal_sys/Subsystem2/Subsystem8 ==
  PosV : Inport
  Pos : Inport  Port=2
  CalibArray : Inport  Port=3
  Delta : Inport  Port=4
  Tolr : Inport  Port=5
  Enable : EnablePort
  XXStIsPos_Get : FunctionCaller  FunctionPrototype=[IsPos,IsPosZone,IsPosAlready] = XXStIsPos_Get(PosV,Pos,CalibArray,Delta,Tolr)  InputArgumentSpecifications=boolean(true), uint16(1), uint16([1;1;1]), uint16(1), uint16(1)  OutputArgumentSpecifications=boolean(true), boolean(true), boolean(true)
  IsPos : Outport
  IsPosZone : Outport  Port=2
  IsPosAlready : Outport  Port=3
  wires:
  XXStIsPos_Get/1 -> IsPos/1
  Pos/1 -> XXStIsPos_Get/2
  Delta/1 -> XXStIsPos_Get/4
  XXStIsPos_Get/3 -> IsPosAlready/1
  PosV/1 -> XXStIsPos_Get/1
  CalibArray/1 -> XXStIsPos_Get/3
  Tolr/1 -> XXStIsPos_Get/5
  XXStIsPos_Get/2 -> IsPosZone/1
